simulink model "system5"  (R2019a)
settings: Solver=ode45  StartTime=0.0  StopTime=10.0  RelTol=1e-9
values from neighbouring files (symbols this model uses):
  beta = 0.001    [Lab3_final.m]
  d_teta0 = 0    [Lab3_final.m]
  g = 9.8    [Lab3_final.m]
  J = m*l^2+(M*L^2)/3    (= 0.00309133333333)    [Lab3_final.m]
  k = 0.35    [Lab3_final.m]
  l = 0.12    [Lab3_final.m]
  L = 0.25    [Lab3_final.m]
  m = 0.07    [Lab3_final.m]
  M = 0.1    [Lab3_final.m]
  teta0 = pi/4    (= 0.785398163397)    [Lab3_final.m]
settings Model: Creator=Vasco  LastModifiedBy=Vasco

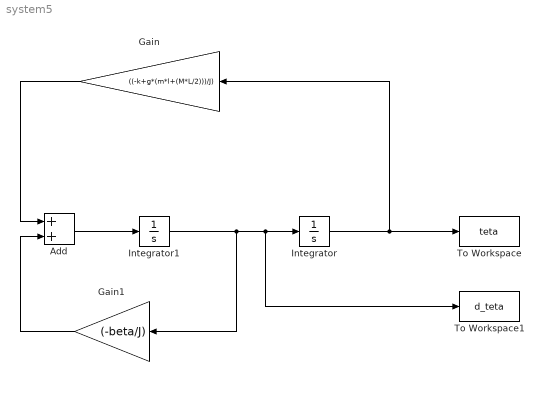
== system system5 ==
  Add : Sum
  Gain : Gain  Gain=((-k+g*(m*l+(M*L/2)))/J)
  Gain1 : Gain  Gain=(-beta/J)
  Integrator : Integrator  InitialCondition=teta0
  Integrator1 : Integrator  InitialCondition=d_teta0
  To Workspace : ToWorkspace  VariableName=teta  SampleTime=-1
      settings: Save2DSignal=2-D array (concatenate along first dimension)
  To Workspace1 : ToWorkspace  VariableName=d_teta  SampleTime=-1
      settings: Save2DSignal=2-D array (concatenate along first dimension)
  wires:
  Integrator1/1 -> Gain1/1, To Workspace1/1, Integrator/1
  Integrator/1 -> Gain/1, To Workspace/1
  Add/1 -> Integrator1/1
  Gain/1 -> Add/1
  Gain1/1 -> Add/2
